simulink model "mot_sim3"  (Simulink 4.00)
settings: Solver=ode45  SolverMode=SingleTasking  StartTime=0.0  StopTime=5  RelTol=1e-3  AbsTol=1e-3
undefined symbols (not defined in the file): b, J, K, L, R
settings Model: LastModifiedBy=R.Babuska  SaveTime=off  SaveOutput=off  LimitDataPoints=off  RTWTemplateMakefile=grt_vc.tmf

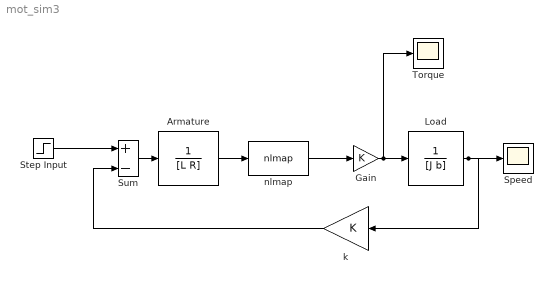
== system mot_sim3 ==
  " k " : Gain  Orientation=left  Gain=K  Multiplication=Element-wise(K.*u)  SaturateOnIntegerOverflow=on
  Armature : TransferFcn  Numerator=1  Denominator=[L R]  AbsoluteTolerance=auto  Realization=auto
  Gain : Gain  Gain=K  Multiplication=Element-wise(K.*u)  SaturateOnIntegerOverflow=on
  Load : TransferFcn  Numerator=1  Denominator=[J b]  AbsoluteTolerance=auto  Realization=auto
  Speed : Scope
      settings: TickLabels=on  TimeRange=auto  YMin=0  YMax=1.5  SaveToWorkspace=off  SaveName=ScopeData  DataFormat=Array  LimitDataPoints=on  MaxDataPoints=5000
  Step Input : Step  Time=1  Before=0  After=40  SampleTime=-1
  Sum : Sum  Inputs=+-  SaturateOnIntegerOverflow=on
  Torque : Scope
      settings: TickLabels=on  TimeRange=auto  YMin=0  YMax=0.2  SaveToWorkspace=off  SaveName=ScopeData  DataFormat=Array  LimitDataPoints=on  MaxDataPoints=5000
  nlmap : MATLABFcn  MATLABFcn=nlmap  OutputDimensions=-1  OutputSignalType=auto  Output1D=on
  wires:
  Load/1 -> Speed/1, " k "/1
  Gain/1 -> Torque/1, Load/1
  nlmap/1 -> Gain/1
  Armature/1 -> nlmap/1
  Sum/1 -> Armature/1
  Step Input/1 -> Sum/1
  " k "/1 -> Sum/2
